simulink model "FeedbackLinearization"  (R2018b)
settings: Solver=FixedStepAuto  StartTime=0.0  StopTime=10  FixedStep=0.01  RelTol=1e-3
libraries: simulink x1
settings Model: Creator=Utente  LastModifiedBy=Utente

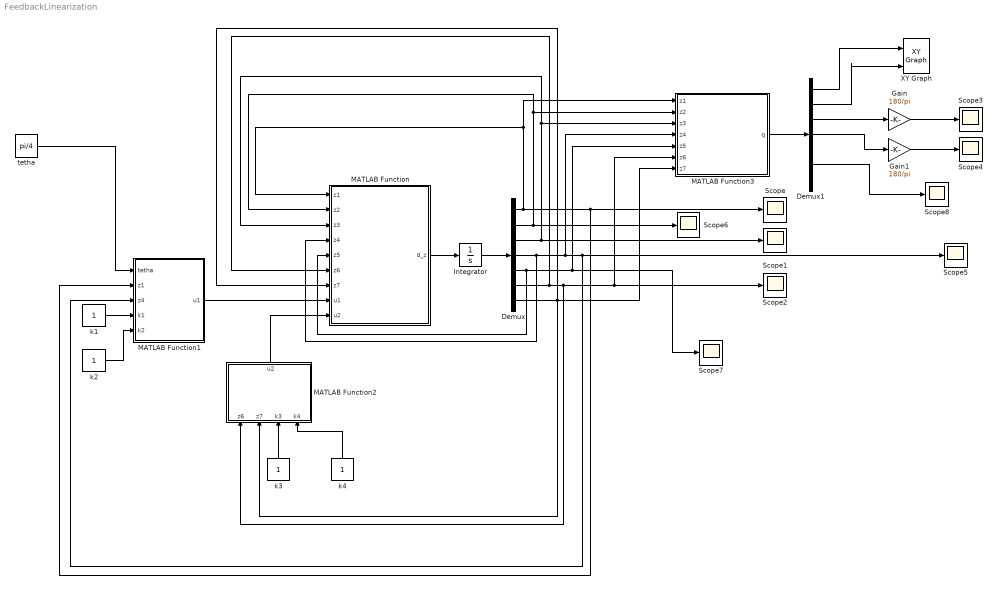
== system FeedbackLinearization ==
  Demux : Demux  Outputs=7
  Demux1 : Demux  Outputs=7
  Gain : Gain  Gain=180/pi
  Gain1 : Gain  Gain=180/pi
  Integrator : Integrator  InitialCondition=[0;0;0;0;0;pi/6;0]
  MATLAB Function : MATLAB Function  TreatAsAtomicUnit=on
  MATLAB Function1 : MATLAB Function  TreatAsAtomicUnit=on
  MATLAB Function2 : MATLAB Function  TreatAsAtomicUnit=on
  MATLAB Function3 : MATLAB Function  TreatAsAtomicUnit=on
  Scope{,1..8} (9 alike) : Scope
  XY Graph : simulink/Sinks/XY Graph  xmin=-100  xmax=100  ymin=-100  ymax=100  st=-1
  k{1..4} (4 alike) : Constant
  "tetha " : Constant  Value=pi/4
  wires:
  MATLAB Function/1(d_z) -> Integrator/1
  Integrator/1 -> Demux/1
  MATLAB Function1/1(u1) -> MATLAB Function/8(u1)
  "tetha "/1 -> MATLAB Function1/1(tetha)
  Demux/4 -> MATLAB Function/4(z4), Scope5/1, MATLAB Function1/3(z4), MATLAB Function3/4(z4)
  k1/1 -> MATLAB Function1/4(k1)
  k2/1 -> MATLAB Function1/5(k2)
  MATLAB Function2/1(u2) -> MATLAB Function/9(u2)
  Demux/6 -> MATLAB Function/6(z6), MATLAB Function3/6(z6), Scope2/1, MATLAB Function2/1(z6)
  Demux/7 -> MATLAB Function3/7(z7), MATLAB Function2/2(z7), MATLAB Function/7(z7)
  k3/1 -> MATLAB Function2/3(k3)
  k4/1 -> MATLAB Function2/4(k4)
  Demux/5 -> MATLAB Function/5(z5), Scope7/1, MATLAB Function3/5(z5)
  Demux/2 -> Scope6/1, MATLAB Function3/2(z2), MATLAB Function/2(z2)
  Demux/1 -> Scope/1, MATLAB Function1/2(z1), MATLAB Function3/1(z1), MATLAB Function/1(z1)
  Demux/3 -> MATLAB Function3/3(z3), MATLAB Function/3(z3), Scope1/1
  MATLAB Function3/1(q) -> Demux1/1
  Demux1/1 -> XY Graph/1
  Demux1/2 -> XY Graph/2
  Demux1/3 -> Gain/1
  Demux1/4 -> Gain1/1
  Gain/1 -> Scope3/1
  Gain1/1 -> Scope4/1
  Demux1/6 -> Scope8/1

== matlab function FeedbackLinearization/MATLAB Function1 ==
  data: tetha input; z1 input; u1 output; z4 input; k1 input; k2 input
function u1 = fcn(tetha,z1,z4,k1,k2)

u1 = -k1*(z1-tetha)-k2*z4;

== matlab function FeedbackLinearization/MATLAB Function ==
  data: z1 input; d_z output; z2 input; z3 input; z4 input; z5 input; z6 input; z7 input; u1 input; u2 input
function d_z = statespace(z1,z2,z3,z4,z5,z6,z7,u1,u2)
        
 
f_f =  [z4; z5 - z3*z4;  z2*z4; 0;
    (sin(2*z6)*((1911*cos(z6)*z4^2)/100000 + 74529/50000) - (1053*z7^2*sin(z6))/25000)/((1521*cos(z6)^2)/10000 - 2619/5000) - (((185367*sin(z6))/5000 + sin(2*z6)*((4753*z4^2)/20000 - (1521*z7^2)/10000))*((39*cos(z6))/1000 + 27/500))/(((39*cos(z6))/100 + 49/10000)*((39*cos(z6)^2)/50 - 2619/5000));
            z7;0];

                                                                                                                                                                                                                                                                                                
g1_f = [0; 0; 0; 1; 0; 0; 0];
g2_f =                                                    [0;
                                                           0;
                                                           0;
                                                           0;
   -((39*cos(z6))/1000 + 27/500)/((39*cos(z6))/100 + 97/200);
                                                           0;
                                                           1];
                                                                                                                                                                                                                                                                                                                                                                                                                                                                                                                                                                                            
d_z = f_f + g1_f*u1 + g2_f*u2;


end

== matlab function FeedbackLinearization/MATLAB Function2 ==
  data: z6 input; u2 output; z7 input; k3 input; k4 input
function u2 = fcn(z6,z7,k3,k4)

    u2 = -k3*z6-k4*z7;

== matlab function FeedbackLinearization/MATLAB Function3 ==
  data: z1 input; q output; z2 input; z3 input; z4 input; z5 input; z6 input; z7 input
function q = transform(z1,z2,z3,z4,z5,z6,z7)

q = zeros(7,1);
A = zeros(2,2);

A = [cos(z1),sin(z1);
     sin(z1),-cos(z1)];

q(1:2,1) = A\[z2;z3];
q(4) = z6;
q(7) = z4;
q(6) = z5;
q(5) = z7;
q(3) = z1;
